simulink model "SET3"  (Simulink 5.0)
settings: Solver=ode45  StartTime=0.0  StopTime=10.0  RelTol=1e-3
settings Model: LastModifiedBy=Administrator

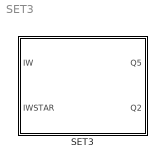
== system SET3 ==
  SET3 : Stateflow chart

== stateflow chart SET3 ==
  settings: updateMethod=CONTINUOUS  executeAtInitialization=1
  state C/
    state C1/
      during:Q5=1;Q2=0;
    state C2/
      during:Q2=1;Q5=0;
    C1 -> C2 : [IW>IWSTAR]
    C2 -> C1 : [IW<IWSTAR]
    (default) -> C1 : [1]
  (default) -> C : [1]
  data: IW input double; IWSTAR input double; Q5 output double; Q2 output double
